simulink model "BasicRobotV2Animation"  (R2023b)
settings: Solver=VariableStepAuto  StartTime=0.0  StopTime=20.0  RelTol=1e-3
values from neighbouring files (symbols this model uses):
  floorsize = 50    [BasicRobot_Parameters.m]
  k_drag = 30    [BasicRobot_Parameters.m]
  m = 2.5    [BasicRobot_Parameters.m]
  r = 0.15    [BasicRobot_Parameters.m]
  rr_collide = 0.05    [BasicRobot_Parameters.m]
  rr_stop = 0.21    [BasicRobot_Parameters.m]
  theta0 = deg2rad(theta0_deg)    [BasicRobot_Parameters.m]
  theta_ref = 1.50    (= 1.5)    [BasicRobot_Parameters.m]
  v_ref = 0.18    [BasicRobot_Parameters.m]
  x_obs = 0    [BasicRobot_Parameters.m]
  y_obs = 0    [BasicRobot_Parameters.m]
undefined symbols (not defined in the file or in its folder): magnitude
libraries: simulink x4, vrlib x2
settings Model: Creator=BeanieBabyJ  LastModifiedBy=BeanieBabyJ

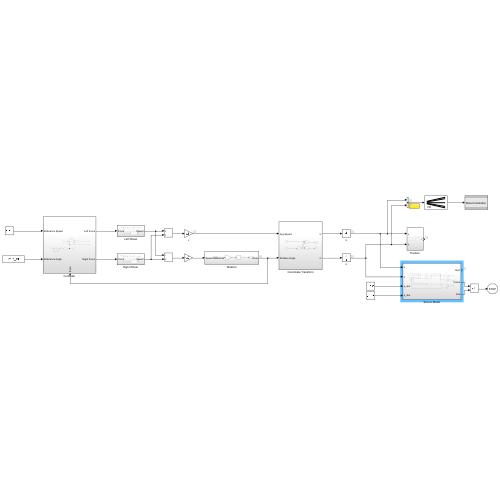
[thumbnail: Simulink's stored preview of the top-level diagram]
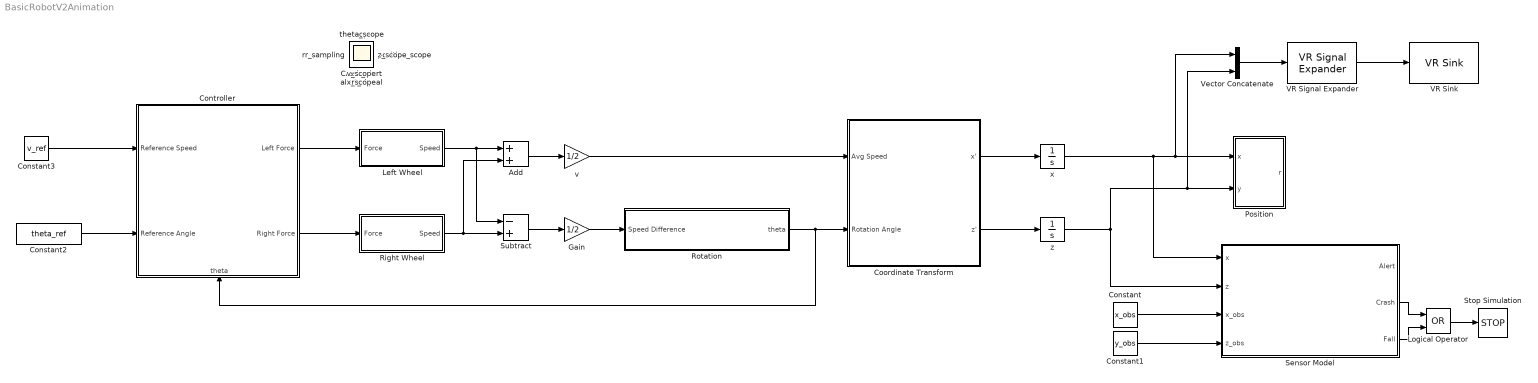
== system BasicRobotV2Animation ==
  Add : Sum
  Constant : Constant  Value=x_obs
  Constant1 : Constant  Value=y_obs
  Constant2 : Constant  Value=theta_ref
  Constant3 : Constant  Value=v_ref
  Controller : Subsystem
      settings: PortSchema="{\"entries\":[{\"content\":{\"sides\":[{\"content\":{\"connectorIds\":[\"In1\",\"In2\"]},\"type\":\"ConnectorPlacement.EquallySpacedRectSide\",\"uuid\":\"ba94545e-9c5b-44f0-b142-601db8af74fa\"},{\"content\":{\"connectorIds\":[\"Out1\",\"Out2\"],\"side\":\"RIGHT\"},\"type\":\"ConnectorPlacement.EquallySpacedRectSide\",\"uuid\":\"af029479-1ae4-4d42-872b-d9816a1308e5\"},{\"content\":{\"side\":\"TOP\"},\"type\":\"ConnectorPlacement.EquallySpacedRectSide\",\"uuid\":\"a7d99619-4318-4ae9-a369-f3fafeea2edf\"},{\"content\":{\"connectorIds\":[\"In3\"],\"side\":\"BOTTOM\"},\"type\":\"ConnectorPlacement.EquallySpacedRectSide\",\"uuid\":\"9d977537-dbbb-45bb-88a3-801d5ac276a0\"}]},\"type\":\"ConnectorPlacement.EquallySpacedConnector\",\"uuid\":\"d5be0c1c-28be-41e4-a0b4-1100c8fad692\"}],\"packageUris\":[\"http://schema.mathworks.com/mf0/Connector/R2020b\"],\"version\":\"1.0\"}"
  Coordinate Transform : Subsystem
  Gain : Gain  Gain=1/2
  Left Wheel : Subsystem
  Logical Operator : Logic  Operator=OR  AllPortsSameDT=off  OutDataTypeStr=boolean
  Position : Subsystem
  Right Wheel : Subsystem
  Rotation : Subsystem
  Sensor Model : Subsystem
  Stop Simulation : Stop
  Subtract : Sum  Inputs=-+
  VR Signal Expander : vrlib/VR Signal Expander  outwidth=3  outidx=[1 3]
  VR Sink : vrlib/VR Sink  InstantiateOnLoad=on  SampleTime=0.1  ViewEnable=on  RemoteChange=off  RemoteView=off  FieldsWritten=Robot.translation.3.1.1.double  WorldFileName=RobotWorld.wrl  AutoView=off  VideoDimensions=[]  AllowVariableSize=off  FigureProperties="{'Position', 'Name', 'Viewpoint', 'CameraBound', 'CameraDirection', 'CameraPosition', 'CameraUpVector', 'ZoomFactor', 'Antialiasing', 'Headlight', 'Lighting', 'NavPanel', 'Sound', 'StatusBar', 'Stereo3D', 'Stereo3DCameraOffset', 'Stereo3DHIT', 'ToolBar', 'Textures', 'Transparency', 'Triad', 'Wireframe', 'NavZones', 'NavMode', 'NavSpeed', 'CaptureFileFormat', 'CaptureFileName', 'Record2DCompressMethod', 'Record2DCompressQuality', 'Record2D', 'Record2DFileName', 'Record2DFPS'; [4.4900000000000000e+02   1.8300000000000000e+02   5.7600000000000000e+02   3.5000000000000000e+02], '', '_untitled_1', 'on', [0.0000000000000000e+00   0.0000000000000000e+00  -1.0000000000000000e+00], [0.0000000000000000e+00   0.0000000000000000e+00   0.0000000000000000e+00], [0.0000000000000000e+00   1.0000000000000000e+00   0.0000000000000000e+00], [1.0000000000000000e+00], 'on', 'on', 'on', 'halfbar', 'on', 'on', 'off', [1.0000000149011612e-01], [0.0000000000000000e+00], 'on', 'on', 'on', 'none', 'off', 'off', 'fly', 'normal', 'tif', '%f_anim_%n.tif', 'auto', [7.5000000000000000e+01], 'off', '%f_anim_%n.avi', 'auto'}"
  Vector Concatenate : Concatenate
  v : Gain  Gain=1/2
  x : Integrator
  z : Integrator
  Crash_alert : Scope
  Scope : Scope
  alert_signal : Scope
  position_scope : Scope
  rr_sampling : Scope
  theta_scope : Scope
  v_scope : Scope
  x_scope : Scope
  z_scope : Scope
  wires:
  Right Wheel/1(Speed) -> Add/2, Subtract/2
  Left Wheel/1(Speed) -> Add/1, Subtract/1
  Subtract/1 -> Gain/1
  Gain/1 -> Rotation/1(Speed Difference)
  Add/1 -> v/1
  v/1 -> Coordinate Transform/1(Avg Speed)
  Controller/2(Right Force) -> Right Wheel/1(Force)
  Coordinate Transform/1(x') -> x/1
  Coordinate Transform/2(z') -> z/1
  Controller/1(Left Force) -> Left Wheel/1(Force)
  x/1 -> Vector Concatenate/1, Position/1(x), Sensor Model/1(x)
  z/1 -> Vector Concatenate/2, Position/2(y), Sensor Model/2(z)
  Constant/1 -> Sensor Model/3(x_obs)
  Constant1/1 -> Sensor Model/4(z_obs)
  Rotation/1(theta) -> Controller/3(theta), Coordinate Transform/2(Rotation Angle)
  Constant2/1 -> Controller/2(Reference Angle)
  Constant3/1 -> Controller/1(Reference Speed)
  VR Signal Expander/1 -> VR Sink/1
  Vector Concatenate/1 -> VR Signal Expander/1
  Sensor Model/2(Crash) -> Logical Operator/1
  Sensor Model/3(Fall) -> Logical Operator/2
  Logical Operator/1 -> Stop Simulation/1

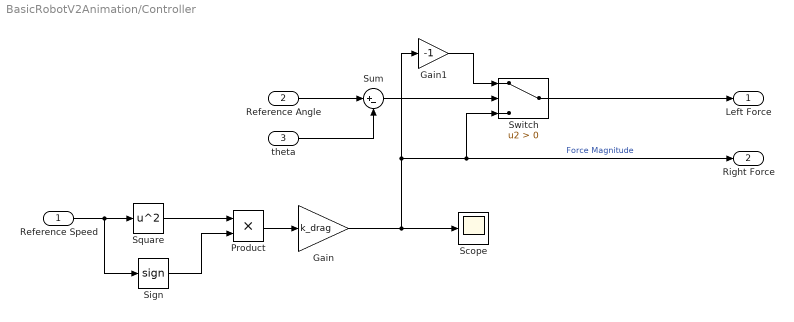
== system BasicRobotV2Animation/Controller ==
  Reference Speed : Inport
  Reference Angle : Inport  Port=2
  theta : Inport  Port=3
  Gain : Gain  Gain=k_drag
  Gain1 : Gain  Gain=-1
  Product : Product
  Scope : Scope
  Sign : Signum
  Square : Math  Operator=square
  Sum : Sum  Inputs=|+-
  Switch : Switch  Criteria=u2 > Threshold  SaturateOnIntegerOverflow=off  InputSameDT=off
  Left Force : Outport
  Right Force : Outport  Port=2
  wires:
  Reference Angle/1 -> Sum/1
  theta/1 -> Sum/2
  Sum/1 -> Switch/2
  Switch/1 -> Left Force/1
  Gain/1 -> Right Force/1, Switch/3, Gain1/1, Scope/1  "Force Magnitude"
  Gain1/1 -> Switch/1
  Reference Speed/1 -> Sign/1, Square/1
  Square/1 -> Product/1
  Sign/1 -> Product/2
  Product/1 -> Gain/1

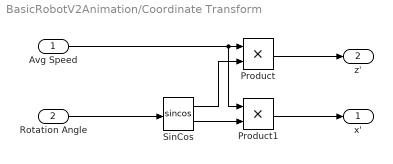
== system BasicRobotV2Animation/Coordinate Transform ==
  Avg Speed : Inport
  Rotation Angle : Inport  Port=2
  Product : Product
  Product1 : Product
  SinCos : Trigonometry  Operator=sincos
  x' : Outport
  z' : Outport  Port=2
  wires:
  Rotation Angle/1 -> SinCos/1
  Avg Speed/1 -> Product1/1, Product/1
  SinCos/1 -> Product/2
  SinCos/2 -> Product1/2
  Product/1 -> z'/1
  Product1/1 -> x'/1

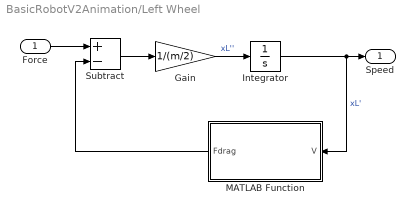
== system BasicRobotV2Animation/Left Wheel ==
  Force : Inport
  Gain : Gain  Gain=1/(m/2)
  Integrator : Integrator
  MATLAB Function : MATLAB Function  TreatAsAtomicUnit=on
  Subtract : Sum  Inputs=+-
  Speed : Outport
  wires:
  Force/1 -> Subtract/1
  MATLAB Function/1(Fdrag) -> Subtract/2
  Subtract/1 -> Gain/1
  Integrator/1 -> MATLAB Function/1(V), Speed/1  "xL'"
  Gain/1 -> Integrator/1  "xL''"

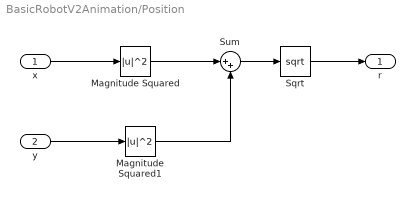
== system BasicRobotV2Animation/Position ==
  x : Inport
  y : Inport  Port=2
  Magnitude Squared : Math  Operator=magnitude^2
  Magnitude Squared1 : Math  Operator=magnitude^2
  Sqrt : Sqrt
  Sum : Sum  Inputs=|++
  r : Outport
  wires:
  Magnitude Squared1/1 -> Sum/2
  Sum/1 -> Sqrt/1
  Magnitude Squared/1 -> Sum/1
  Sqrt/1 -> r/1
  x/1 -> Magnitude Squared/1
  y/1 -> Magnitude Squared1/1

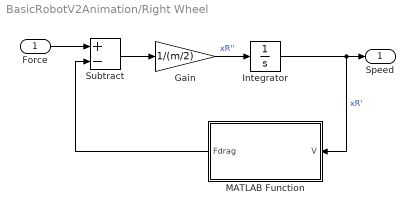
== system BasicRobotV2Animation/Right Wheel ==
  Force : Inport
  Gain : Gain  Gain=1/(m/2)
  Integrator : Integrator
  MATLAB Function : MATLAB Function  TreatAsAtomicUnit=on
  Subtract : Sum  Inputs=+-
  Speed : Outport
  wires:
  Integrator/1 -> MATLAB Function/1(V), Speed/1  "xR'"
  Gain/1 -> Integrator/1  "xR''"
  Force/1 -> Subtract/1
  MATLAB Function/1(Fdrag) -> Subtract/2
  Subtract/1 -> Gain/1

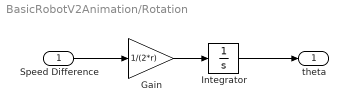
== system BasicRobotV2Animation/Rotation ==
  Speed Difference : Inport
  Gain : Gain  Gain=1/(2*r)
  Integrator : Integrator  InitialCondition=theta0
  theta : Outport
  wires:
  Speed Difference/1 -> Gain/1
  Gain/1 -> Integrator/1
  Integrator/1 -> theta/1

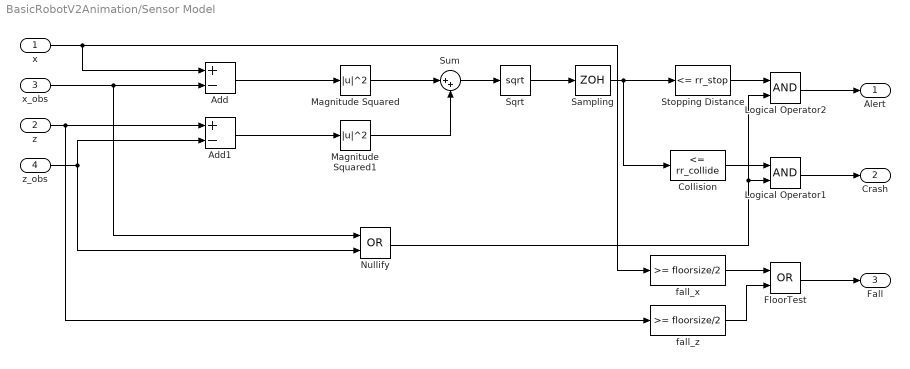
== system BasicRobotV2Animation/Sensor Model ==
  x : Inport
  z : Inport  Port=2
  x_obs : Inport  Port=3
  z_obs : Inport  Port=4
  Add : Sum  Inputs=+-
  Add1 : Sum  Inputs=+-
  Collision : simulink/Logic and Bit Operations/Compare To Constant  relop=<=  const=rr_collide  OutDataTypeStr=boolean
  FloorTest : Logic  Operator=OR  AllPortsSameDT=off  OutDataTypeStr=boolean
  Logical Operator1 : Logic  AllPortsSameDT=off  OutDataTypeStr=boolean
  Logical Operator2 : Logic  AllPortsSameDT=off  OutDataTypeStr=boolean
  Magnitude Squared : Math  Operator=magnitude^2
  Magnitude Squared1 : Math  Operator=magnitude^2
  Nullify : Logic  Operator=OR  AllPortsSameDT=off  OutDataTypeStr=boolean
  Sampling : ZeroOrderHold  SampleTime=0.25
  Sqrt : Sqrt
  Stopping Distance : simulink/Logic and Bit Operations/Compare To Constant  relop=<=  const=rr_stop  OutDataTypeStr=boolean
  Sum : Sum  Inputs=|++
  fall_x : simulink/Logic and Bit Operations/Compare To Constant  relop=>=  const=floorsize/2  OutDataTypeStr=boolean
  fall_z : simulink/Logic and Bit Operations/Compare To Constant  relop=>=  const=floorsize/2  OutDataTypeStr=boolean
  Alert : Outport
  Crash : Outport  Port=2
  Fall : Outport  Port=3
  wires:
  Sampling/1 -> Collision/1, Stopping Distance/1
  x/1 -> fall_x/1, Add/1
  Magnitude Squared/1 -> Sum/1
  Sum/1 -> Sqrt/1
  Add/1 -> Magnitude Squared/1
  Add1/1 -> Magnitude Squared1/1
  Sqrt/1 -> Sampling/1
  x_obs/1 -> Nullify/1, Add/2
  z/1 -> fall_z/1, Add1/1
  z_obs/1 -> Nullify/2, Add1/2
  Magnitude Squared1/1 -> Sum/2
  Collision/1 -> Logical Operator1/1
  Logical Operator1/1 -> Crash/1
  Nullify/1 -> Logical Operator2/2, Logical Operator1/2
  Stopping Distance/1 -> Logical Operator2/1
  Logical Operator2/1 -> Alert/1
  fall_x/1 -> FloorTest/1
  FloorTest/1 -> Fall/1
  fall_z/1 -> FloorTest/2

== matlab function BasicRobotV2Animation/Right Wheel/MATLAB Function ==
  data: Fdrag output; V input; k_drag parameter
function Fdrag=get_fdrag(V, k_drag)

Fdrag=k_drag*V*abs(V);

== matlab function BasicRobotV2Animation/Left Wheel/MATLAB Function ==
  data: Fdrag output; V input; k_drag parameter
function Fdrag=get_fdrag(V, k_drag)

Fdrag=k_drag*V*abs(V);
